simulink model "VR_BESS_Kalman_2018"  (R2018a)
settings: Solver=ode23tb  StartTime=0.0  StopTime=0.8  MaxStep=1e-05  RelTol=1e-3
undefined symbols (not defined in the file or in its folder): Acid, Lead
libraries: powerlib x17, electricdrivelib x1
settings Model: Creator=valac  LastModifiedBy=Admin
settings SolverCC: ZeroCrossControl=DisableAll  ZeroCrossAlgorithm=Adaptive
settings DataIOCC: ReturnWorkspaceOutputs=on
settings SFSimCC: SimUseLocalCustomCode=on
settings RTWCC: RTWUseLocalCustomCode=on

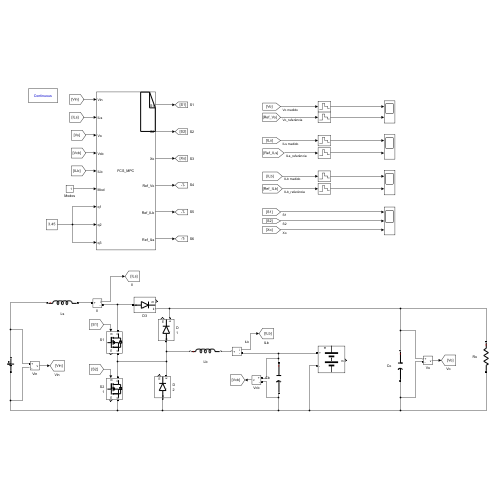
[thumbnail: Simulink's stored preview of the top-level diagram]
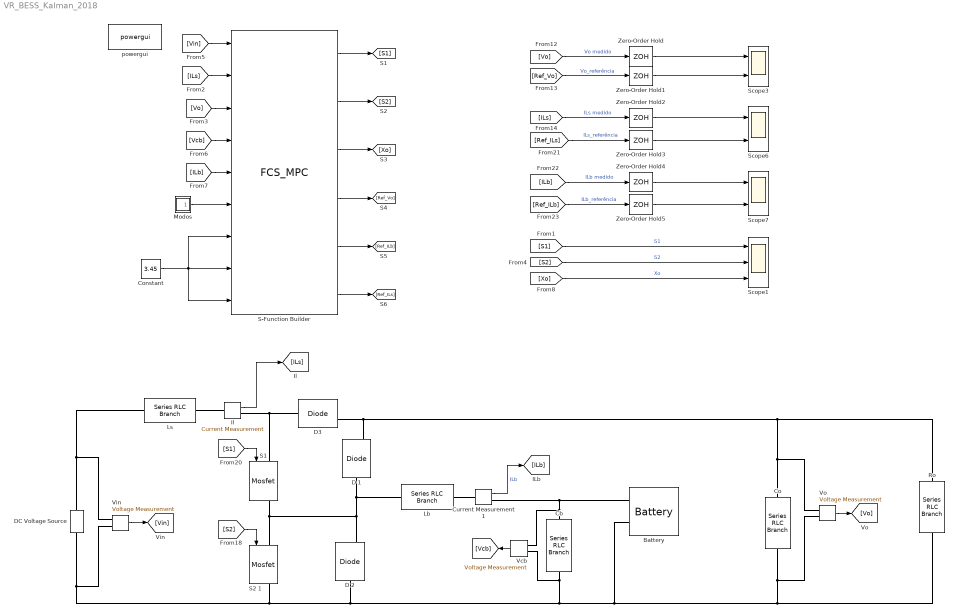
== system VR_BESS_Kalman_2018 ==
  Battery : electricdrivelib/Extra Sources/Battery  BatType=Lead-Acid  ShowTempParam=off  ThermalPreset=no  ShowAgeParam=off  NomV=120  NomQ=5.4  SOC=90  Batt_Tr=0.03  PresetModel=off  MaxQ=5.625  MinV=90  FullV=130.6579  Dis_rate=7  R=0.01  Normal_OP=1.6755  expZone="[122.1711         0.018]"  current=[6.5 13 32.5]  Units=Time  Tci=20  NomT=20  T2=-30  MaxQ2=4.8  FullV2=7.1  Normal_OP2=5.655  expZone2="[6.58           1]"  Rca=0.6  ti=2000  Dp=0  Neq0=0  Tsim=1e6  Ta1=25  Qeol=5.4*0.9  Reol=0.013333*1.2  Char_age=[2.3478, 3]  Dis_age=[2.3478, 10]  N1=1500  N2=10500  N3=1000  N4=1400  Ta2=45  N5=950
  Cb : powerlib/Elements/Series RLC Branch  LConnTagsString=__new0  RConnTagsString=__new0  BranchType=C  Resistance=0.01  Inductance=1e-3  SetiL0=off  InitialCurrent=0  Capacitance=500e-6  Setx0=on  InitialVoltage=120  Measurements=None
  Co : powerlib/Elements/Series RLC Branch  LConnTagsString=__new0  RConnTagsString=__new0  BranchType=C  Resistance=1  Inductance=1e-3  SetiL0=off  InitialCurrent=0  Capacitance=400e-6  Setx0=on  InitialVoltage=400  Measurements=None
  Constant : Constant  Value=3.45
  Current Measurement1 : powerlib/Measurements/Current Measurement  PhasorSimulation=off  OutputType=Complex  PSBequivalent=0
  D 1 : powerlib/Power Electronics/Diode  Ron=0.001  Lon=0  Vf=0.8  IC=0  UseSnubber=0  Rs=inf  Cs=250e-9  Measurements=on
  D 2 : powerlib/Power Electronics/Diode  Ron=0.001  Lon=0  Vf=0.8  IC=0  UseSnubber=0  Rs=inf  Cs=250e-9  Measurements=on
  "D3 " : powerlib/Power Electronics/Diode  Ron=0.001  Lon=0  Vf=0.8  IC=0  UseSnubber=0  Rs=inf  Cs=250e-9  Measurements=on
  DC Voltage Source : powerlib/Electrical Sources/DC Voltage Source  Amplitude=300  Measurements=None
  "Il " : powerlib/Measurements/Current Measurement  PhasorSimulation=off  OutputType=Complex  PSBequivalent=0
  Lb : powerlib/Elements/Series RLC Branch  LConnTagsString=__new0  RConnTagsString=__new0  BranchType=L  Resistance=1  Inductance=3e-3  SetiL0=on  InitialCurrent=1.08  Capacitance=1e-6  Setx0=off  InitialVoltage=0  Measurements=None
  Ls : powerlib/Elements/Series RLC Branch  LConnTagsString=__new0  RConnTagsString=__new0  BranchType=L  Resistance=1  Inductance=3.5e-3  SetiL0=on  InitialCurrent=3.5  Capacitance=1e-6  Setx0=off  InitialVoltage=0  Measurements=None
  Modos : Subsystem
  Ro : powerlib/Elements/Series RLC Branch  LConnTagsString=__new0  RConnTagsString=__new0  BranchType=R  Resistance=160  Inductance=1e-3  SetiL0=off  InitialCurrent=0  Capacitance=1e-6  Setx0=off  InitialVoltage=0  Measurements=None
  S-Function Builder : S-Function  InitFcn=try, set_param(gcb,'FunctionName','FCS_MPC'), end  FunctionName=FCS_MPC  SFunctionModules=FCS_MPC_wrapper.cpp  SFunctionDeploymentMode=off  EnableBusSupport=off  mask(S-Function Builder){}
      mask help: Simulink:masks:SFunctionBuilder_MD
      mask init:
      | val = [[.9  0.75 0.75 1 1 .9 .9 1]',[1 1 0.75 0.75 .9 .9 1 .9]'];try , sys = get_param(gcb,'SfunBuilderFcnName');if isempty(sys), sys = get_param(gcb,'FunctionName'); end,catch, sys = get_param(gcb,'FunctionName'); end
      settings: CopyFcn=set_param(gcbh,'LinkStatus','none')  PreSaveFcn=try, set_param(gcb,'FunctionName','FCS_MPC'), end  OpenFcn=sfunctionwizard(gcbh)
      mask Display:
      | plot(val(:,1),val(:,2))
      | disp(sys)
      | port_label('input',1,sprintf('%s', 'Vin'),'interpreter','tex')
      | port_label('input',2,sprintf('%s', 'ILs'),'interpreter','tex')
      | port_label('input',3,sprintf('%s', 'Vo'),'interpreter','tex')
      | port_label('input',4,sprintf('%s', 'Vcb'),'interpreter','tex')
      | port_label('input',5,sprintf('%s', 'ILb'),'interpreter','tex')
      | port_label('input',6,sprintf('%s', 'Mod'),'interpreter','tex')
      | port_label('input',7,sprintf('%s', 'q1'),'interpreter','tex')
      | port_label('input',8,sprintf('%s', 'q2'),'interpreter','tex')
      | port_label('input',9,sprintf('%s', 'q3'),'interpreter','tex')
      | port_label('output',1,sprintf('%s', 'S1'),'interpreter','tex')
      | port_label('output',2,sprintf('%s', 'S2'),'interpreter','tex')
      | port_label('output',3,sprintf('%s', 'Xo'),'interpreter','tex')
      | port_label('output',4,sprintf('%s', 'Ref\_Vo'),'interpreter','tex')
      | port_label('output',5,sprintf('%s', 'Ref\_ILb'),'interpreter','tex')
      | port_label('output',6,sprintf('%s', 'Ref\_ILs'),'interpreter','tex')
  "S1 " : powerlib/Power Electronics/Mosfet  Ron=0.001  Lon=0  Rd=0.00000000001  Vfd=0  IC=0  Rs=1e5  Cs=inf  Measurements=on
  S2 1 : powerlib/Power Electronics/Mosfet  Ron=0.001  Lon=0  Rd=0.00000000001  Vfd=0  IC=0  Rs=1e5  Cs=inf  Measurements=on
  Scope1 : Scope  NumInputPorts=3
  Scope3 : Scope  NumInputPorts=2
  Scope6 : Scope  NumInputPorts=2
  Scope7 : Scope  NumInputPorts=2
  Vcb : powerlib/Measurements/Voltage Measurement  PhasorSimulation=off  OutputType=Complex  PSBequivalent=0
  Vin : powerlib/Measurements/Voltage Measurement  PhasorSimulation=off  OutputType=Complex  PSBequivalent=0
  "Vo " : powerlib/Measurements/Voltage Measurement  PhasorSimulation=off  OutputType=Complex  PSBequivalent=0
  Zero-Order Hold{,1..5} (6 alike) : ZeroOrderHold  SampleTime=1/100e3
  powergui : powerlib/powergui  Priority=1  SimulationMode=Continuous  SampleTime=1/100e+05  frequency=60  Iterations=50  frequencyindice=0  Pbase=100e6  ErrMax=1e-4  UnitsV=kV  UnitsW=MW  buscounter=0  FunctionMessages=off  echomessages=off  EnableUseOfTLC=off  CurrentSourceSwitches=off  DisableSnubberDevices=off  DisableRonSwitches=off  DisableVfSwitches=off  DisplayEquations=off  AutomaticDiscreteSolvers=off  SolverType=Tustin/Backward Euler (TBE)  Interpol=off  ExternalGateDelay=off  methode=off  Ts=100  x0status=blocks  SPID=on  SwTol=0  HookPort=off  NonlinearTolerance=1e-4  nMaxIteration=100  ContinueOnMaxIteration=off  RestoreLinks=warning  ResistiveCurrentMeasurement=off  Frange=[0:2:500]  Ylog=off  Xlog=on  ShowGrid=off  save=off  variable=ZData  structure=0  ZoomFFT=off  StartTime=0.0  cycles=1  DisplayStyle=1  fundamental=60  FreqAxis=off  MaxFrequency=1000  frequencyindicesteady=1  RmsSteady=1  display=off
  wires:
  Vcb/1 -> [Vcb]
  Vin/1 -> [Vin]
  S-Function Builder/1 -> [S1]
  S-Function Builder/2 -> [S2]
  [Vin] -> S-Function Builder/1
  [Vcb] -> S-Function Builder/4
  [ILb] -> S-Function Builder/5
  [ILs] -> S-Function Builder/2
  [Vo] -> S-Function Builder/3
  [S1] -> "S1 "/1
  [S2] -> S2 1/1
  S-Function Builder/3 -> [Xo]
  Current Measurement1/1 -> [ILb]  "ILb"
  S-Function Builder/4 -> [Ref_Vo]
  S-Function Builder/6 -> [Ref_ILs]
  S-Function Builder/5 -> [Ref_ILb]
  [Vo] -> Zero-Order Hold/1  "Vo medido"
  [Ref_Vo] -> Zero-Order Hold1/1  "Vo_referência"
  [ILs] -> Zero-Order Hold2/1  "ILs medido"
  [Ref_ILs] -> Zero-Order Hold3/1  "ILs_referência"
  [ILb] -> Zero-Order Hold4/1  "ILb medido"
  [Ref_ILb] -> Zero-Order Hold5/1  "ILb_referência"
  "Il "/1 -> [ILs]
  "Vo "/1 -> [Vo]
  Constant/1 -> S-Function Builder/7, S-Function Builder/9, S-Function Builder/8
  Modos/1(Out1) -> S-Function Builder/6
  [S2] -> Scope1/2  "S2"
  [S1] -> Scope1/1  "S1"
  [Xo] -> Scope1/3  "Xo"
  Zero-Order Hold/1 -> Scope3/1
  Zero-Order Hold1/1 -> Scope3/2
  Zero-Order Hold2/1 -> Scope6/1
  Zero-Order Hold3/1 -> Scope6/2
  Zero-Order Hold4/1 -> Scope7/1
  Zero-Order Hold5/1 -> Scope7/2
  connections:
  D 2/LConn1 -- Battery/LConn2 -- Ro/RConn1 -- Co/RConn1 -- "Vo "/LConn2 -- Vcb/LConn2 -- Cb/RConn1 -- DC Voltage Source/LConn1 -- Vin/LConn2 -- S2 1/RConn1
  Lb/LConn1 -- D 2/RConn1 -- S2 1/LConn1 -- "S1 "/RConn1 -- D 1/LConn1
  "Vo "/LConn1 -- Co/LConn1 -- Ro/LConn1 -- D 1/RConn1 -- "D3 "/RConn1
  "S1 "/LConn1 -- "Il "/RConn1 -- "D3 "/LConn1
  Ls/RConn1 -- "Il "/LConn1
  Current Measurement1/RConn1 -- Battery/LConn1 -- Vcb/LConn1 -- Cb/LConn1
  Current Measurement1/LConn1 -- Lb/RConn1
  Vin/LConn1 -- DC Voltage Source/RConn1 -- Ls/LConn1

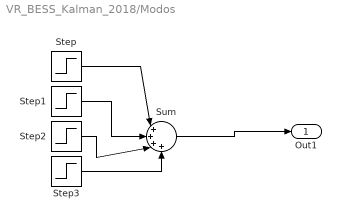
== system VR_BESS_Kalman_2018/Modos ==
  Step : Step  Time=0  Before=1  SampleTime=0
  Step1 : Step  Time=0.2  SampleTime=0
  Step2 : Step  Time=0.4  SampleTime=0
  Step3 : Step  Time=0.6  SampleTime=0
  Sum : Sum  Inputs=|++++
  Out1 : Outport
  wires:
  Step1/1 -> Sum/2
  Step/1 -> Sum/1
  Step2/1 -> Sum/3
  Step3/1 -> Sum/4
  Sum/1 -> Out1/1
